simulink model "lab4_model52"  (R2020b)
settings: Solver=VariableStepAuto  StartTime=0.0  StopTime=7  RelTol=1e-3
settings Model: Creator=mluser  LastModifiedBy=mluser

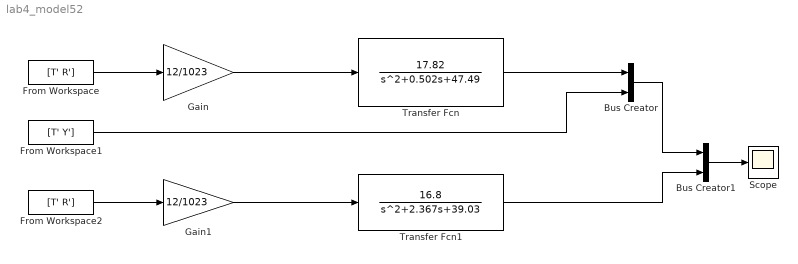
== system lab4_model52 ==
  Bus Creator : BusCreator  Inputs=2
  Bus Creator1 : BusCreator  Inputs=2
  From Workspace : FromWorkspace  VariableName=[T' R']  SampleTime=0.002
  From Workspace1 : FromWorkspace  VariableName=[T' Y']  SampleTime=0.002
  From Workspace2 : FromWorkspace  VariableName=[T' R']  SampleTime=0.002
  Gain : Gain  Gain=12/1023
  Gain1 : Gain  Gain=12/1023
  Scope : Scope
  Transfer Fcn : TransferFcn  Numerator=[17.82]  Denominator=[1 0.502 47.49]
  Transfer Fcn1 : TransferFcn  Numerator=[16.8]  Denominator=[1 2.367 39.03]
  wires:
  Gain/1 -> Transfer Fcn/1
  Transfer Fcn/1 -> Bus Creator/1
  From Workspace/1 -> Gain/1
  From Workspace1/1 -> Bus Creator/2
  From Workspace2/1 -> Gain1/1
  Gain1/1 -> Transfer Fcn1/1
  Transfer Fcn1/1 -> Bus Creator1/2
  Bus Creator/1 -> Bus Creator1/1
  Bus Creator1/1 -> Scope/1
